simulink library "FMmodelBasic"  (R2022b)
settings: Solver=ode45  StartTime=0.0  StopTime=10.0  RelTol=1e-3  EnableMultiTasking=on
undefined symbols (not defined in the file or in its folder): aeroDB, envDB
libraries: utils x1
(part 2 of 2)

== matlab function FMmodelBasic/LSA_02_Fmmodel/aircraft/2_output_variables_part1/22_coordinate_transformations/221_geodetic_to_bodyfixed/Tfg ==
  data: r8x3attitude input; r8T_fg output
function r8T_fg = trans_fg(r8x3attitude)

r8phi = r8x3attitude(1);
r8th = r8x3attitude(2);
r8psi = r8x3attitude(3);

r8T_fg = [cos(r8th)*cos(r8psi) cos(r8th)*sin(r8psi) -sin(r8th)
    ((sin(r8phi)*sin(r8th))-(cos(r8phi)*sin(r8psi))) ((sin(r8phi)*sin(r8th))+(cos(r8phi)*cos(r8psi))) (sin(r8phi)*cos(r8th))
    (cos(r8phi)*sin(r8th)*cos(r8psi))+(sin(r8phi)*sin(r8psi)) (cos(r8phi)*sin(r8th)*sin(r8psi))-(sin(r8phi)*cos(r8psi)) (cos(r8phi)*cos(r8th))];

== matlab function FMmodelBasic/LSA_02_Fmmodel/integrationProcces/Vec2Bus XT ==
  data: vec input; bu_Xaircraft output Bus: bu_Xaircraft
function bu_Xaircraft = vec2busXmotion(vec)

bu_Xaircraft.bu_XmotionEq.r8x3om_f = zeros(3,1);
bu_Xaircraft.bu_XmotionEq.r8x3attitude = zeros(3,1);
bu_Xaircraft.bu_XmotionEq.r8x3VK_f = zeros(3,1);
bu_Xaircraft.bu_XmotionEq.r8x3rCG0_g = zeros(3,1);

bu_Xaircraft.bu_XmotionEq.r8x3om_f(1,1)= vec(1);
bu_Xaircraft.bu_XmotionEq.r8x3om_f(2,1)= vec(2);
bu_Xaircraft.bu_XmotionEq.r8x3om_f(3,1)= vec(3);
bu_Xaircraft.bu_XmotionEq.r8x3attitude(1,1)= vec(4);
bu_Xaircraft.bu_XmotionEq.r8x3attitude(2,1)= vec(5);
bu_Xaircraft.bu_XmotionEq.r8x3attitude(3,1)= vec(6);
bu_Xaircraft.bu_XmotionEq.r8x3VK_f(1,1)= vec(7);
bu_Xaircraft.bu_XmotionEq.r8x3VK_f(2,1)= vec(8);
bu_Xaircraft.bu_XmotionEq.r8x3VK_f(3,1)= vec(9);
bu_Xaircraft.bu_XmotionEq.r8x3rCG0_g(1,1)= vec(10);
bu_Xaircraft.bu_XmotionEq.r8x3rCG0_g(2,1)= vec(11);
bu_Xaircraft.bu_XmotionEq.r8x3rCG0_g(3,1)= vec(12);

end

== matlab function FMmodelBasic/LSA_02_Fmmodel/aircraft/2_output_variables_part1/23_flightpath/MATLAB Function ==
  data: r8x3VK_g input; r8VK output; r8ga output; r8Ch output
function [r8VK,r8ga,r8Ch] = VKGamCalc(r8x3VK_g)
[az,elev,r] = cart2sph(r8x3VK_g(1),r8x3VK_g(2),r8x3VK_g(3));
r8VK = r;
r8ga = -elev;
r8Ch = az;

== matlab function FMmodelBasic/LSA_02_Fmmodel/aircraft/4_environment/41_atmosphere/412_wind/4121_windVelocity_g/MATLAB Function ==
  data: r8gaW input; r8x3VW_g output size=[3,1]; r8ChW input; r8VW input
function r8x3VW_g = VwCalc(r8gaW,r8ChW,r8VW)
[uwg,vwg,wwg] = sph2cart(r8ChW,-r8gaW,r8VW);
r8x3VW_g = [uwg;vwg;wwg];
end

== matlab function FMmodelBasic/LSA_02_Fmmodel/aircraft/5_aerodynamics/51_effective_flow_at_ARP/512_flow_angles_and_airspeed/MATLAB Function ==
  data: r8x3VAARP_f input; r8alARP output; r8beARP output; r8VAARP output
function [r8alARP,r8beARP,r8VAARP] = alBeCalc(r8x3VAARP_f)
[r8beARP,r8alARP,r8VAARP] = cart2sph(r8x3VAARP_f(1),r8x3VAARP_f(2),r8x3VAARP_f(3));
end

== matlab function FMmodelBasic/LSA_02_Fmmodel/aircraft/5_aerodynamics/52_wing_and_fuselage/521_influence_variables/MATLAB Function ==
  data: r8x3om_f input; r8VAARP input; r8p1 output; aeroDB parameter; r8q1 output; r8r1 output
function [r8p1,r8q1,r8r1] = rotationalVelCalc(r8x3om_f,r8VAARP,aeroDB)

r8p1 = r8x3om_f(1)*aeroDB.b*0.5/r8VAARP;
r8q1 = r8x3om_f(2)*aeroDB.lmu/r8VAARP;
r8r1 = r8x3om_f(3)*aeroDB.b*0.5/r8VAARP;
